simulink model "quatquad_sim"  (R2021b)
settings: Solver=FixedStepAuto  StartTime=0.0  StopTime=tsim  FixedStep=Ts  RelTol=1e-3
settings Model: Creator=vifre  LastModifiedBy=vifre

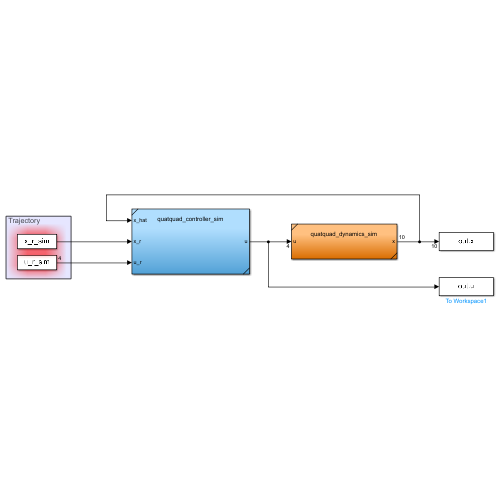
[thumbnail: Simulink's stored preview of the top-level diagram]
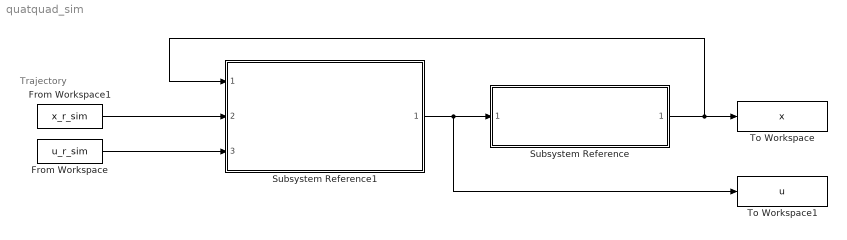
== system quatquad_sim ==
  note: Trajectory
  From Workspace : FromWorkspace  VariableName=u_r_sim
  From Workspace1 : FromWorkspace  VariableName=x_r_sim
  Subsystem Reference : Subsystem  ReferencedSubsystem=quatquad_dynamics_sim
  Subsystem Reference1 : Subsystem  ReferencedSubsystem=quatquad_controller_sim
  To Workspace : ToWorkspace  VariableName=x  SampleTime=-1
      settings: Save2DSignal=2-D array (concatenate along first dimension)
  To Workspace1 : ToWorkspace  VariableName=u  SampleTime=-1
      settings: Save2DSignal=2-D array (concatenate along first dimension)
  wires:
  Subsystem Reference/1 -> To Workspace/1, Subsystem Reference1/1
  From Workspace/1 -> Subsystem Reference1/3
  Subsystem Reference1/1 -> To Workspace1/1, Subsystem Reference/1
  From Workspace1/1 -> Subsystem Reference1/2
